simulink model "Ejemplo_3_2"  (R2013a)
settings: Solver=ode45  StartTime=0.0  StopTime=10.0  RelTol=1e-3
settings Model: Creator=Miguel  LastModifiedBy=Miguel

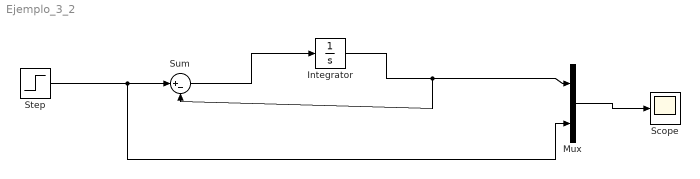
== system Ejemplo_3_2 ==
  Integrator : Integrator
  Mux : Mux  Inputs=2
  Scope : Scope
      settings: ShowLegends=on
  Step : Step  SampleTime=0
  Sum : Sum  Inputs=|+-
  wires:
  Integrator/1 -> Sum/2, Mux/1
  Mux/1 -> Scope/1
  Step/1 -> Mux/2, Sum/1
  Sum/1 -> Integrator/1
